simulink model "lab1_model"  (Simulink 7.9)
settings: Solver=ode45  StartTime=0.0  StopTime=10.0  RelTol=1e-3
values from neighbouring files (symbols this model uses):
  cpw = 4190    [skrypt.m]    (also in symulacja_dyn.m = cpw_; testerka.m)
  Cvg = cpw*row*Vg    (= 410620)    [skrypt.m]    (also in symulacja_dyn.m = cpw*row*Vg)
  Cvw = cpp*rop*Vp    (= 89586)    [skrypt.m]    (also in symulacja_dyn.m = cpp*rop*Vp)
  dFg = 0    [skrypt.m]    (also in symulacja_dyn.m = dFg_; testerka.m)
  dQt = dQt_    [symulacja_dyn.m]    (also in testerka.m = 0)
  dTgz = 0    [skrypt.m]    (also in symulacja_dyn.m = dTgz_; testerka.m)
  dTzew = dTzew_    [symulacja_dyn.m]    (also in testerka.m = 0)
  Fg_0 = Fg_n    (= 0.000243534167844)    [skrypt.m]    (also in symulacja_dyn.m = Fg_n)
  kg = Q_n/(Tgsr_n-Twew_n)    (= 400)    [skrypt.m]    (also in symulacja_dyn.m = Q_n/(Tgsr_n-Twew_n))
  kw = (Q_n-Qt_n)/(Twew_n-Tzew_n)    (= 500)    [skrypt.m]    (also in symulacja_dyn.m = (Q_n-Qt_0)/(Twew_n-Tzew_n))
  Qt_0 = 0    [symulacja_dyn.m]
  row = 980    [skrypt.m]    (also in symulacja_dyn.m = row_; testerka.m)
  Tgp_n = 70    [skrypt.m]    (also in symulacja_dyn.m = Tgp_n_; testerka.m)
  Tgz_0 = Tgz_n    (= 90)    [skrypt.m]    (also in symulacja_dyn.m = Tgz_n)
  Twew_n = 20    [skrypt.m]    (also in symulacja_dyn.m = Twew_n_; testerka.m)
  Tzew_0 = Tzew_n    (= -20)    [skrypt.m]    (also in symulacja_dyn.m = Tzew_n)
settings Model: Creator=LAB320-1537-User  LastModifiedBy=LAB320-1537-User

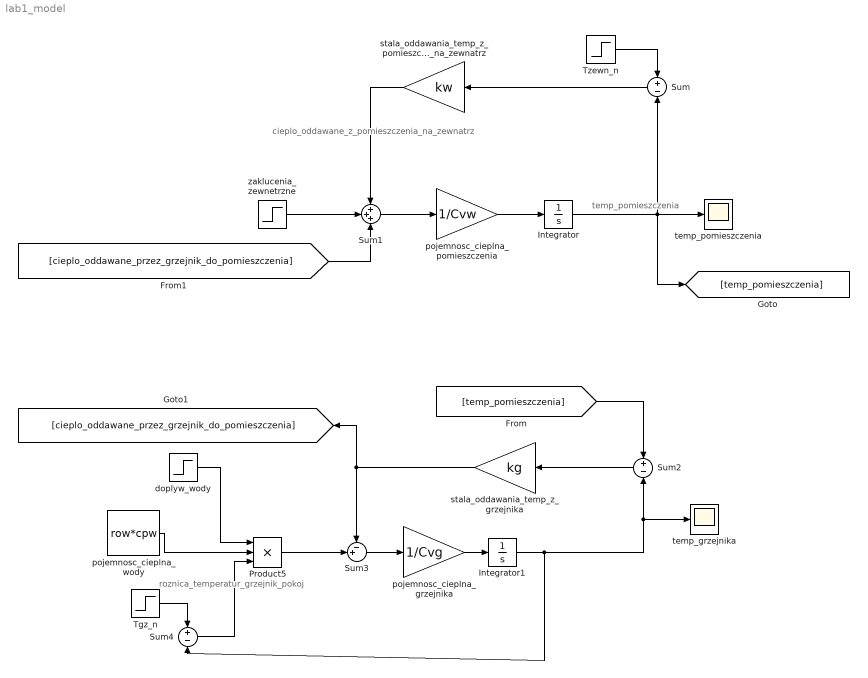
== system lab1_model ==
  note: cieplo_oddawane_z_pomieszczenia_na_zewnatrz
  note: temp_pomieszczenia
  note: roznica_temperatur_grzejnik_pokoj
  Integrator : Integrator  InitialCondition=Twew_n
  Integrator1 : Integrator  InitialCondition=Tgp_n
  Product5 : Product  Inputs=3  RndMeth=Zero
  Sum : Sum  Inputs=+-
  Sum1 : Sum  Inputs=+++
  Sum2 : Sum  Inputs=+-
  Sum3 : Sum  Inputs=-+|
  Sum4 : Sum  Inputs=+-
  Tgz_n : Step  Before=Tgz_0  After=Tgz_0+dTgz  SampleTime=0
  Tzewn_n : Step  Before=Tzew_0  After=Tzew_0+dTzew  SampleTime=0
  doplyw_wody : Step  Before=Fg_0  After=Fg_0+dFg  SampleTime=0
  pojemnosc_cieplna_grzejnika : Gain  Gain=1/Cvg
  pojemnosc_cieplna_pomieszczenia : Gain  Gain=1/Cvw
  pojemnosc_cieplna_wody : Constant  Value=row*cpw
  stala_oddawania_temp_z_grzejnika : Gain  Gain=kg
  stala_oddawania_temp_z_pomieszczenia_na_zewnatrz : Gain  Gain=kw
  temp_grzejnika : Scope
  temp_pomieszczenia : Scope
  zaklucenia_zewnetrzne : Step  Before=Qt_0  After=Qt_0+dQt  SampleTime=0
  wires:
  Tzewn_n/1 -> Sum/1
  Integrator1/1 -> temp_grzejnika/1, Sum2/2, Sum4/2
  Product5/1 -> Sum3/2
  doplyw_wody/1 -> Product5/1
  stala_oddawania_temp_z_grzejnika/1 -> Sum3/1, [cieplo_oddawane_przez_grzejnik_do_pomieszczenia]
  Integrator/1 -> temp_pomieszczenia/1, Sum/2, [temp_pomieszczenia]
  Tgz_n/1 -> Sum4/1
  Sum4/1 -> Product5/3
  pojemnosc_cieplna_wody/1 -> Product5/2
  Sum1/1 -> pojemnosc_cieplna_pomieszczenia/1
  pojemnosc_cieplna_pomieszczenia/1 -> Integrator/1
  Sum2/1 -> stala_oddawania_temp_z_grzejnika/1
  Sum3/1 -> pojemnosc_cieplna_grzejnika/1
  pojemnosc_cieplna_grzejnika/1 -> Integrator1/1
  Sum/1 -> stala_oddawania_temp_z_pomieszczenia_na_zewnatrz/1
  stala_oddawania_temp_z_pomieszczenia_na_zewnatrz/1 -> Sum1/1
  [temp_pomieszczenia] -> Sum2/1
  zaklucenia_zewnetrzne/1 -> Sum1/2
  [cieplo_oddawane_przez_grzejnik_do_pomieszczenia] -> Sum1/3
